simulink model "HydrostaticCVTTestHarness"  (R2025a)
settings: Solver=daessc  StartTime=0.0  StopTime=8  RelTol=1e-3
PostLoadFcn:
  | hydrostaticCVT.displacementPump= 60;
  | hydrostaticCVT.shaftVelocityNominal= 1800;
  | hydrostaticCVT.nominalPressureGain=10;
  | hydrostaticCVT.efficiencyVolumetric= 0.9700;
  | hydrostaticCVT.efficiencyMechanical= 0.9200;
  | hydrostaticCVT.displacementMotor= 180;
  | hydrostaticCVT.displacementPumpAux= 5;
  | hydrostaticCVT.shaftVelocityNominalAux= 1000;
  | hydrostaticCVT.gearRatioAux= 10;
  | hydrostaticCVT.pressDifferentialCracking= 0.0300;
  | hydrostaticCVT.pressDifferentialMaxOpen= 0.1000;
  | hydrostaticCVT.areaMax= 1.0000e-05;
  | hydrostaticCVT.areaLeak= 1.0000e-10;
  | hydrostaticCVT.cd= 0.6500;
  | hydrostaticCVT.pressDifferentialSet= 25;
  | hydrostaticCVT.pressRegulationRange= 0.3500;
  | hydrostaticCVT.maxArea= 2.0000e-05;
  | hydrostaticCVT.pressDifferentialSetAux= 1;
  | hydrostaticCVT.pressRegulationRangeAux= 0.1500;
  | hydrostaticCVT.lengthPipe= 2;
  | hydrostaticCVT.diameterPipe= 0.0500;
libraries: fl_lib x9, sdl_lib x2, nesl_utility x1
CloseFcn:
  | clear hydrostaticCVT;
settings Model: Creator=asakhare  LastModifiedBy=varora
settings SolverCC: MaxConsecutiveMinStep=10
settings SimscapeCC: SimscapeLogType=all

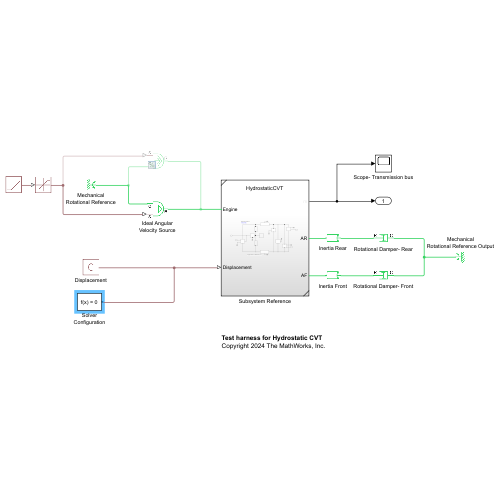
[thumbnail: Simulink's stored preview of the top-level diagram]
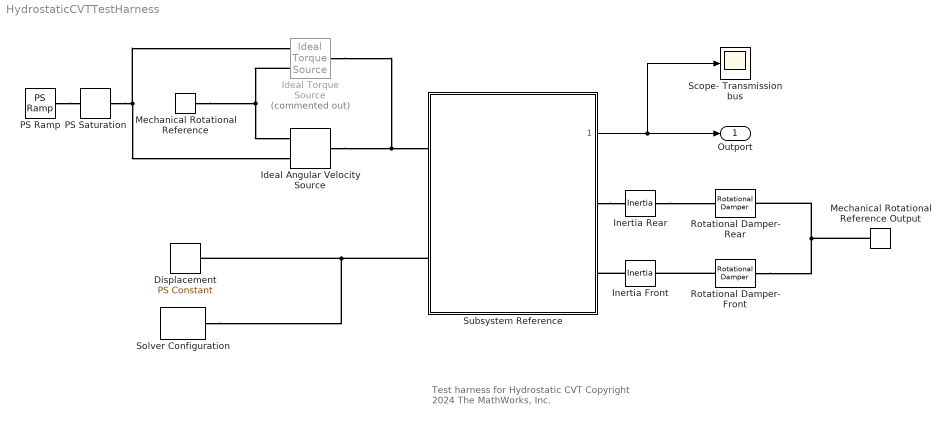
== system HydrostaticCVTTestHarness ==
  note: Test harness for Hydrostatic CVT
      | Copyright 2024 The MathWorks, Inc.
  Displacement : fl_lib/Physical Signals/Sources/PS Constant  constant=60 cm^3/rev
  Ideal Angular Velocity Source : fl_lib/Mechanical/Mechanical Sources/Ideal Angular Velocity Source
  Ideal Torque Source : fl_lib/Mechanical/Mechanical Sources/Ideal Torque Source  Commented=on
  Inertia Front : fl_lib/Mechanical/Rotational Elements/Inertia  inertia=0.01 kg*m^2  num_ports=foundation.enum.numPorts2.two  w_specify=off  w_priority=High  w=0 rad/s  w_nominal_specify=off  w_nominal_value=1  w_nominal_unit=rad/s  t_specify=off  t_priority=None  t=0 N*m  t_nominal_specify=off  t_nominal_value=1  t_nominal_unit=N*m
      settings: InternalSimscapePortConfiguration="{\"Bottom\":[],\"Left\":[{\"id\":\"I\",\"label\":\"\",\"type\":\"foundation.mechanical.rotational.rotational\"}],\"Right\":[{\"id\":\"J\",\"label\":\"\",\"type\":\"foundation.mechanical.rotational.rotational\"}],\"Top\":[]}"
  Inertia Rear : fl_lib/Mechanical/Rotational Elements/Inertia  inertia=0.01 kg*m^2  num_ports=foundation.enum.numPorts2.two  w_specify=off  w_priority=High  w=0 rad/s  w_nominal_specify=off  w_nominal_value=1  w_nominal_unit=rad/s  t_specify=off  t_priority=None  t=0 N*m  t_nominal_specify=off  t_nominal_value=1  t_nominal_unit=N*m
      settings: InternalSimscapePortConfiguration="{\"Bottom\":[],\"Left\":[{\"id\":\"I\",\"label\":\"\",\"type\":\"foundation.mechanical.rotational.rotational\"}],\"Right\":[{\"id\":\"J\",\"label\":\"\",\"type\":\"foundation.mechanical.rotational.rotational\"}],\"Top\":[]}"
  Mechanical Rotational Reference : fl_lib/Mechanical/Rotational Elements/Mechanical Rotational Reference
  Mechanical Rotational Reference Output : fl_lib/Mechanical/Rotational Elements/Mechanical Rotational Reference
  PS Ramp : fl_lib/Physical Signals/Sources/PS Ramp  slope=200 rpm/s  start_time=0.5 s  initial_output=0 rpm  ZeroCross=true
  PS Saturation : fl_lib/Physical Signals/Nonlinear Operators/PS Saturation  upper_limit=500 rpm  lower_limit=0 rpm  ZeroCross=true
  Rotational Damper- Front : sdl_lib/Couplings & Drives/Springs & Dampers/Rotational Damper  D=1 N*m*s/rad  thermal_port=simscape.enum.thermaleffects.omit  thermal_mass=50 kJ/K  temperature_specify=off  temperature_priority=High  temperature=300 K  temperature_nominal_specify=off  temperature_nominal_value=1  temperature_nominal_unit=K
  Rotational Damper- Rear : sdl_lib/Couplings & Drives/Springs & Dampers/Rotational Damper  D=1 N*m*s/rad  thermal_port=simscape.enum.thermaleffects.omit  thermal_mass=50 kJ/K  temperature_specify=off  temperature_priority=High  temperature=300 K  temperature_nominal_specify=off  temperature_nominal_value=1  temperature_nominal_unit=K
  Scope- Transmission bus : Scope
      settings: ActiveDisplayYMinimum=-10.55928  ActiveDisplayYMaximum=91.45501
  Solver Configuration : nesl_utility/Solver Configuration  PhysicalDomain=network_engine_domain  SubClassName=solver  LeftPortType=input  RightPortType=generic  Tones=[]  Harmonics=[]  SimulateNoise=off  Profile=off  UseLocalSampling=off  EnableSwitchedLinearOptims=on  FrequencyDomain=off  UseCCode=off  RelTol=0.001  AbsTol=0.001  MinStep=1e-09  ToWorkspace=off  RevertToSquareIcSolve=off  NumHomotopyIterations=100  PhasorMode=off  PhasorModeNumHarmonics=1  ConsistencySolver=NEWTON_XTOL_AFTER_FTOL  IndexReductionMethod=DerivativeReplacement  DoDC=off  ResidualTolerance=1e-09  ConsistencyTolSource=GLOBAL  ConsistencyAbsTol=0.001  ConsistencyRelTol=0.001  ConsistencyTolFactor=0.001  UseLocalSolver=off  LocalSolverChoice=NE_BACKWARD_EULER_ADVANCER  ResolveIndetEquations=on  FunctionEvalNumThread=1  LocalSolverSampleTime=0.001  DoFixedCost=off  MaxNonlinIter=3  MaxModeIter=2  ComputeImpulses=off  ImpulseIterations=2  LinearAlgebra=auto  LinearAlgebraNumThread=0  EquationFormulation=NE_TIME_EF  DelaysMemoryBudget=1024  AutomaticFiltering=on  FilteringTimeConstant=0.001  PartitionStorageMethod=AS_NEEDED  PartitionMemoryBudget=1024  PartitionMethod=ROBUST  MultibodyUseLocalSolver=off  MultibodyLocalSolverChoice=ODE1  MultibodyLocalSolverSampleTime=0.001
  Subsystem Reference : Subsystem  ReferencedSubsystem=HydrostaticCVT
  Outport : Outport
  wires:
  Subsystem Reference/1 -> Scope- Transmission bus/1, Outport/1
  connections:
  Ideal Angular Velocity Source/LConn1 -- Ideal Torque Source/LConn1 -- Subsystem Reference/LConn1
  Mechanical Rotational Reference/LConn1 -- Ideal Torque Source/RConn2 -- Ideal Angular Velocity Source/RConn2
  Subsystem Reference/LConn2 -- Solver Configuration/RConn1 -- Displacement/RConn1
  Rotational Damper- Front/LConn1 -- Inertia Front/LConn1
  Subsystem Reference/RConn1 -- Inertia Rear/RConn1
  Mechanical Rotational Reference Output/LConn1 -- Rotational Damper- Front/RConn1 -- Rotational Damper- Rear/RConn1
  Inertia Front/RConn1 -- Subsystem Reference/RConn2
  Inertia Rear/LConn1 -- Rotational Damper- Rear/LConn1
  PS Ramp/RConn1 -- PS Saturation/LConn1
  PS Saturation/RConn1 -- Ideal Torque Source/RConn1 -- Ideal Angular Velocity Source/RConn1
